simulink model "przestrzen_stanu_2"  (R2014b)
settings: Solver=ode45  StartTime=0.0  StopTime=10.0  RelTol=1e-3
values from neighbouring files (symbols this model uses):
  A2 = [ - den_z(2:end); 1 0 0; 0 1 0 ]'    [zad_2.m]
  B2 = [ num_z(2:end)' ]    [zad_2.m]
undefined symbols (not defined in the file or in its folder): Tp, x0
settings Model: Creator=Konrad  LastModifiedBy=Konrad

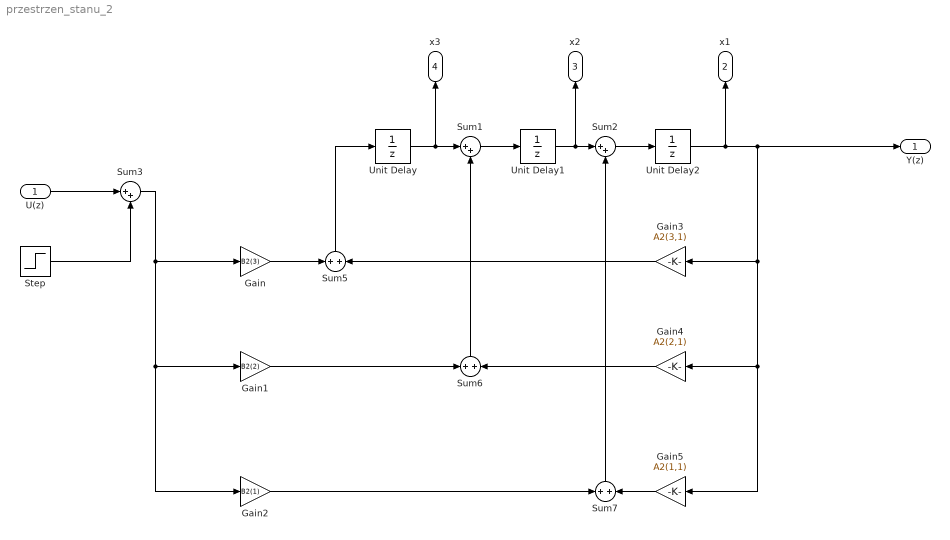
== system przestrzen_stanu_2 ==
  U(z) : Inport
  Gain : Gain  Gain=B2(3)
  Gain1 : Gain  Gain=B2(2)
  Gain2 : Gain  Gain=B2(1)
  Gain3 : Gain  Gain=A2(3,1)
  Gain4 : Gain  Gain=A2(2,1)
  Gain5 : Gain  Gain=A2(1,1)
  Step : Step  SampleTime=0
  Sum1 : Sum  Inputs=|++
  Sum2 : Sum  Inputs=|++
  Sum3 : Sum  Inputs=|++
  Sum5 : Sum  Inputs=+|+
  Sum6 : Sum  Inputs=+|+
  Sum7 : Sum  Inputs=+|+
  Unit Delay : UnitDelay  InitialCondition=x0(3)  SampleTime=Tp
  Unit Delay1 : UnitDelay  InitialCondition=x0(2)  SampleTime=Tp
  Unit Delay2 : UnitDelay  InitialCondition=x0(1)  SampleTime=Tp
  Y(z) : Outport
  x1 : Outport  Port=2
  x2 : Outport  Port=3
  x3 : Outport  Port=4
  wires:
  Sum1/1 -> Unit Delay1/1
  Unit Delay1/1 -> x2/1, Sum2/1
  Sum2/1 -> Unit Delay2/1
  Unit Delay/1 -> x3/1, Sum1/1
  Gain/1 -> Sum5/1
  Unit Delay2/1 -> x1/1, Y(z)/1, Gain3/1, Gain4/1, Gain5/1
  Gain3/1 -> Sum5/2
  Gain4/1 -> Sum6/2
  Gain5/1 -> Sum7/2
  Gain1/1 -> Sum6/1
  Gain2/1 -> Sum7/1
  Sum6/1 -> Sum1/2
  Sum7/1 -> Sum2/2
  Sum3/1 -> Gain/1, Gain1/1, Gain2/1
  Sum5/1 -> Unit Delay/1
  U(z)/1 -> Sum3/1
  Step/1 -> Sum3/2
